simulink model "simu4_lqr"  (R2024a)
settings: Solver=VariableStepAuto  StartTime=0.0  StopTime=10  RelTol=1e-3
settings Model: Creator=Soyann805  LastModifiedBy=psp_dada

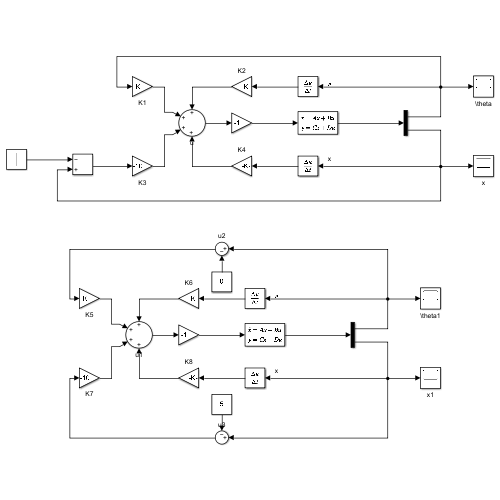
[thumbnail: Simulink's stored preview of the top-level diagram]
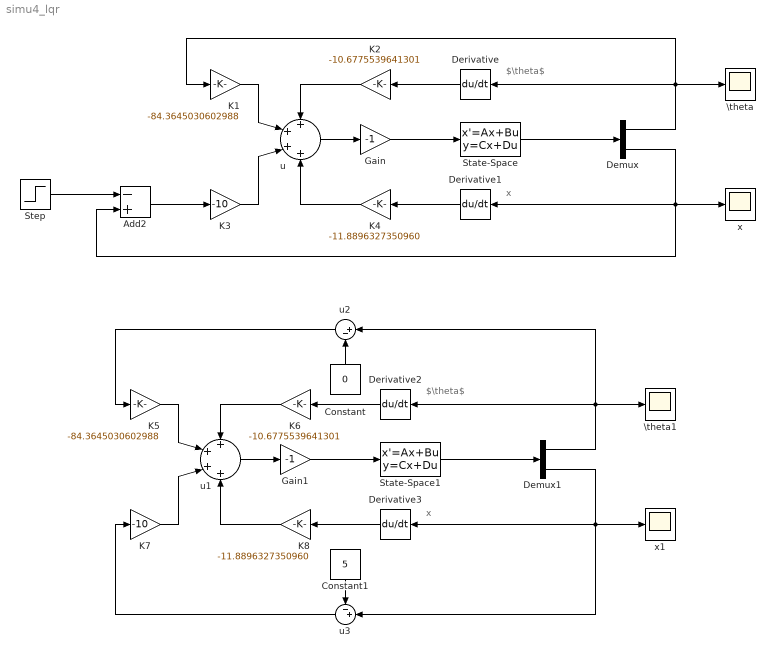
== system simu4_lqr ==
  note: $\theta$
  note: x
  note: $\theta$
  note: x
  Add2 : Sum  Inputs=-+
  Constant : Constant  Value=0
  Constant1 : Constant  Value=5
  Demux : Demux  Outputs=2
  Demux1 : Demux  Outputs=2
  Derivative{,1..3} (4 alike) : Derivative
  Gain : Gain  Gain=-1
  Gain1 : Gain  Gain=-1
  K1 : Gain  Gain=-84.3645030602988
  K2 : Gain  Gain=-10.6775539641301
  K3 : Gain  Gain=-10
  K4 : Gain  Gain=-11.8896327350960
  K5 : Gain  Gain=-84.3645030602988
  K6 : Gain  Gain=-10.6775539641301
  K7 : Gain  Gain=-10
  K8 : Gain  Gain=-11.8896327350960
  State-Space : StateSpace  A=[0 1 0 0; 41.6300 0 0 0; 0 0 0 1;-0.6099 0 0 0];  B=[0;-2.7584;0;0.6898]  C=[1 0 0 0;0 0 1 0]  D=[0;0]  InitialCondition=[2 0 3 0]
  State-Space1 : StateSpace  A=[0 1 0 0; 41.6300 0 0 0; 0 0 0 1;-0.6099 0 0 0];  B=[0;-2.7584;0;0.6898]  C=[1 0 0 0;0 0 1 0]  D=[0;0]  InitialCondition=[2 0 3 0]
  Step : Step  Time=0  After=-0.5  SampleTime=0
  \theta : Scope
  \theta1 : Scope
  u : Sum  Inputs=++++
  u1 : Sum  Inputs=++++
  u2 : Sum  Inputs=|+-
  u3 : Sum  Inputs=-+|
  x : Scope
  x1 : Scope
  wires:
  K1/1 -> u/2
  K2/1 -> u/1
  K3/1 -> u/3
  K4/1 -> u/4
  Demux/2 -> x/1, Derivative1/1, Add2/2
  u/1 -> Gain/1
  State-Space/1 -> Demux/1
  Demux/1 -> K1/1, \theta/1, Derivative/1
  Derivative/1 -> K2/1
  Step/1 -> Add2/1
  Add2/1 -> K3/1
  Derivative1/1 -> K4/1
  Gain/1 -> State-Space/1
  K6/1 -> u1/1
  Demux1/1 -> u2/1, \theta1/1, Derivative2/1
  Demux1/2 -> u3/2, x1/1, Derivative3/1
  Gain1/1 -> State-Space1/1
  State-Space1/1 -> Demux1/1
  K5/1 -> u1/2
  K7/1 -> u1/3
  K8/1 -> u1/4
  u1/1 -> Gain1/1
  Derivative3/1 -> K8/1
  Derivative2/1 -> K6/1
  Constant1/1 -> u3/1
  Constant/1 -> u2/2
  u2/1 -> K5/1
  u3/1 -> K7/1
